simulink model "SimPrac7"  (R2018a)
settings: Solver=ode45  StartTime=0.0  StopTime=20  RelTol=1e-9
values from neighbouring files (symbols this model uses):
  K1 = 2    [Prac7.m]
  K2 = 1    [Prac7.m]
  K3 = 1    [Prac7.m]
  Kdif = 1    [Prac7.m]
  Kg = Kfg*Kwg*Kag*Rng    [Prac7.m]
  Kint = 1    [Prac7.m]
  Kreg = 2    [Prac7.m]
  T1g = Tfg+ Tag    [Prac7.m]
  T2g = (Tfg*Tag)^0.5    [Prac7.m]
  Tf1 = 10    [Prac7.m]
  Tf2 = 4    [Prac7.m]
  Ung = 110    [Prac7.m]
settings Model: Creator=dirlak  LastModifiedBy=dirlak

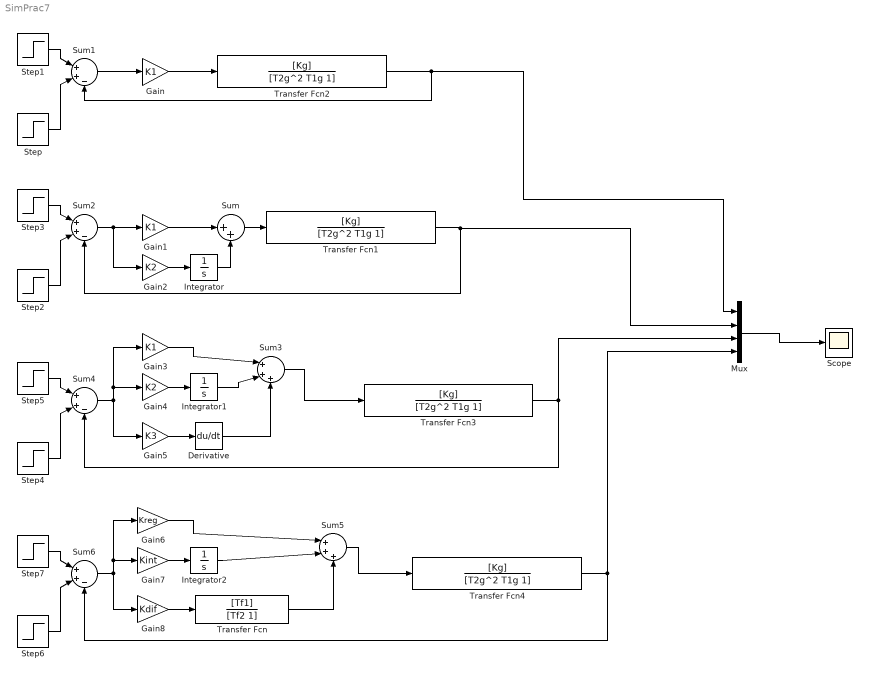
== system SimPrac7 ==
  Derivative : Derivative
  Gain : Gain  Gain=K1
  Gain1 : Gain  Gain=K1
  Gain2 : Gain  Gain=K2
  Gain3 : Gain  Gain=K1
  Gain4 : Gain  Gain=K2
  Gain5 : Gain  Gain=K3
  Gain6 : Gain  Gain=Kreg
  Gain7 : Gain  Gain=Kint
  Gain8 : Gain  Gain=Kdif
  Integrator : Integrator
  Integrator1 : Integrator
  Integrator2 : Integrator
  Mux : Mux
  Scope : Scope
  Step{,2,4,6} (4 alike) : Step  Time=10  After=Ung  SampleTime=0
  Step{1,3,5,7} (4 alike) : Step  Time=0  After=Ung  SampleTime=0
  Sum : Sum  Inputs=|++
  Sum{1..2,4,6} (4 alike) : Sum  Inputs=|++-
  Sum3 : Sum  Inputs=|+++
  Sum5 : Sum  Inputs=|+++
  Transfer Fcn : TransferFcn  Numerator=[Tf1]  Denominator=[Tf2 1]
  Transfer Fcn{1..4} (4 alike) : TransferFcn  Numerator=[Kg]  Denominator=[T2g^2 T1g 1]
  wires:
  Sum1/1 -> Gain/1
  Transfer Fcn2/1 -> Mux/1, Sum1/3
  Gain/1 -> Transfer Fcn2/1
  Step1/1 -> Sum1/1
  Step/1 -> Sum1/2
  Sum2/1 -> Gain2/1, Gain1/1
  Step3/1 -> Sum2/1
  Step2/1 -> Sum2/2
  Gain1/1 -> Sum/1
  Sum/1 -> Transfer Fcn1/1
  Gain2/1 -> Integrator/1
  Integrator/1 -> Sum/2
  Integrator1/1 -> Sum3/2
  Transfer Fcn3/1 -> Mux/3, Sum4/3
  Sum3/1 -> Transfer Fcn3/1
  Step4/1 -> Sum4/2
  Sum4/1 -> Gain5/1, Gain3/1, Gain4/1
  Step5/1 -> Sum4/1
  Gain4/1 -> Integrator1/1
  Gain3/1 -> Sum3/1
  Gain5/1 -> Derivative/1
  Derivative/1 -> Sum3/3
  Gain8/1 -> Transfer Fcn/1
  Gain7/1 -> Integrator2/1
  Gain6/1 -> Sum5/1
  Integrator2/1 -> Sum5/2
  Sum6/1 -> Gain8/1, Gain6/1, Gain7/1
  Transfer Fcn4/1 -> Mux/4, Sum6/3
  Step6/1 -> Sum6/2
  Sum5/1 -> Transfer Fcn4/1
  Step7/1 -> Sum6/1
  Transfer Fcn/1 -> Sum5/3
  Mux/1 -> Scope/1
  Transfer Fcn1/1 -> Mux/2, Sum2/3
